simulink model "model_breach"  (R2019b)
settings: Solver=VariableStepAuto  StartTime=0.0  StopTime=nb_time_unit_in_a_simulation/5  RelTol=1e-3
values from neighbouring files (symbols this model uses):
  nb_air_cons = nb_rooms-2    [load_parameters.m]
  nb_boilers = 2    [load_parameters.m]
  nb_radiators = nb_rooms-2    [load_parameters.m]
  nb_second_in_timeunit = 60*5    (= 300)    [full_test.m]
  nb_step_to_fifteen_min = 3    [full_test.m]
  nb_step_to_one_h = 12    [full_test.m]
  nb_step_to_thirty_min = 6    [full_test.m]
  timeunit_in_a_day = 2*6*24    (= 288)    [full_test.m]
undefined symbols (not defined in the file or in its folder): air_mass_kg_rooms, Area_boiler, area_outdoor_rooms, Area_radiators, area_rooms_ground, area_walls_between_rooms, C_air, C_water, Energy_used_by_air_conditioner_for_1_timeunit_in_Watts_vector, Energy_used_by_air_mixer_for_1_timeunit_in_Watts, Energy_used_by_boiler_for_1_timeunit_in_Watts, initial_relative_humidity, initial_temp_water_in_boilers, initial_temperature_rooms, initial_temperature_water_in_radiator, k_boiler_border, k_radiators, k_wall_outdoor_rooms, k_walls_between_rooms, mass_water_radiator, matrix_AC_rooms_locations, matrix_boiler_radiator_connection, matrix_boiler_rooms_locations, matrix_radiator_rooms_locations, nb_humans, nb_rooms, outdoor_max_temp_A, outdoor_max_temp_B, outdoor_min_temp_A, outdoor_min_temp_B, tau_boiler, thickness_boiler, thickness_outdoor_rooms, thickness_radiator_pipes, thickness_walls_between_rooms, Volume_radiators, Volume_rooms, water_weight_in_boiler, watt_generation_of_employe
libraries: dspmtrx3 x15, slstlib x6, dspstat3 x6, simulink x2
(part 2 of 2)

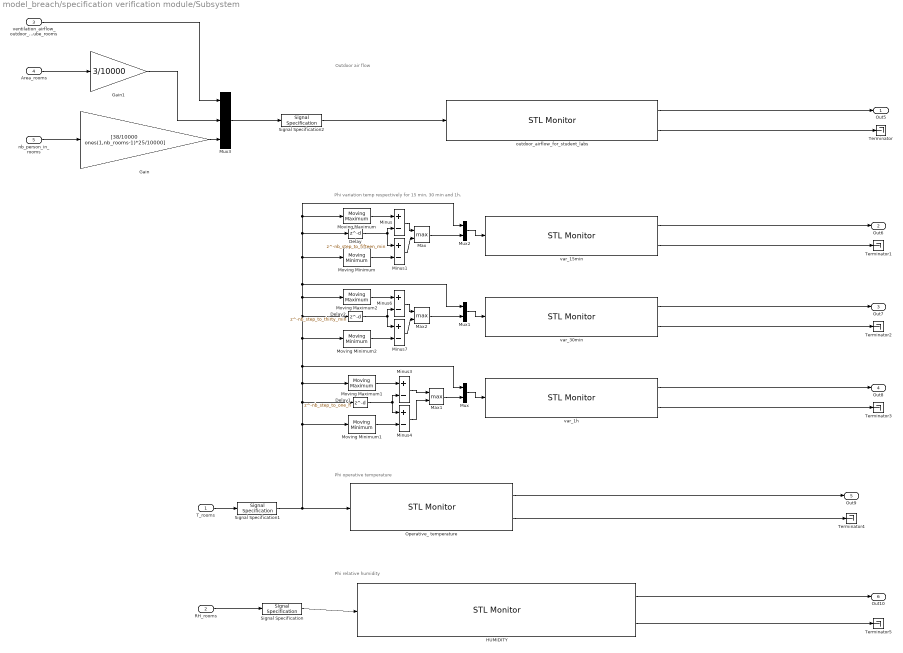
== system model_breach/specification verification module/Subsystem ==
  note: Phi variation temp respectively for 15 min, 30 min and 1h.
  note: Outdoor air flow
  note: Phi operative temperature
  note: Phi relative humidity
  T_rooms : Inport  PortDimensions=nb_rooms
  RH_rooms : Inport  Port=2  PortDimensions=nb_rooms
  ventilation_airflow_outdoor_air_mcube_rooms : Inport  Port=3  PortDimensions=nb_rooms
  Area_rooms : Inport  Port=4  PortDimensions=nb_rooms
  nb_person_in_rooms : Inport  Port=5  OutDataTypeStr=double  PortDimensions=nb_rooms
  Delay : Delay  DelayLength=nb_step_to_fifteen_min  InitialCondition=27
  Delay1 : Delay  DelayLength=nb_step_to_one_h  InitialCondition=27
  Delay2 : Delay  DelayLength=nb_step_to_thirty_min  InitialCondition=27
  Gain : Gain  Gain=[38/10000 ones(1,nb_rooms-1)*25/10000]
  Gain1 : Gain  Gain=3/10000
  "HUMIDITY " : slstlib/STL Monitor  SignalNames=name_rh  STLString=formula_rh  MaxRob=1  RefreshRate=rate  rob_low_lim=inf  rob_up_lim=-inf  rob_diff_lim=-inf
      settings: SourceProductName=Breach Library
  Max : MinMax  Function=max  Inputs=2  ZeroCross=off
  Max1 : MinMax  Function=max  Inputs=2  ZeroCross=off
  Max2 : MinMax  Function=max  Inputs=2  ZeroCross=off
  Minus{,1,3..4,6..7} (6 alike) : Sum  Inputs=+-
  Moving Maximum : dspstat3/Moving Maximum  SpecifyWindowLength=on  WindowLength=nb_step_to_fifteen_min  SimulateUsing=Code generation
      settings: SourceProductName=DSP System Toolbox  SourceProductBaseCode=DS
  Moving Maximum1 : dspstat3/Moving Maximum  SpecifyWindowLength=on  WindowLength=nb_step_to_one_h  SimulateUsing=Code generation
      settings: SourceProductName=DSP System Toolbox  SourceProductBaseCode=DS
  Moving Maximum2 : dspstat3/Moving Maximum  SpecifyWindowLength=on  WindowLength=nb_step_to_thirty_min  SimulateUsing=Code generation
      settings: SourceProductName=DSP System Toolbox  SourceProductBaseCode=DS
  Moving Minimum : dspstat3/Moving Minimum  SpecifyWindowLength=on  WindowLength=nb_step_to_fifteen_min  SimulateUsing=Code generation
      settings: SourceProductName=DSP System Toolbox  SourceProductBaseCode=DS
  Moving Minimum1 : dspstat3/Moving Minimum  SpecifyWindowLength=on  WindowLength=nb_step_to_one_h  SimulateUsing=Code generation
      settings: SourceProductName=DSP System Toolbox  SourceProductBaseCode=DS
  Moving Minimum2 : dspstat3/Moving Minimum  SpecifyWindowLength=on  WindowLength=nb_step_to_thirty_min  SimulateUsing=Code generation
      settings: SourceProductName=DSP System Toolbox  SourceProductBaseCode=DS
  Mux : Mux  Inputs=2
  Mux1 : Mux  Inputs=2
  Mux2 : Mux  Inputs=2
  Mux3 : Mux  Inputs=[nb_rooms nb_rooms nb_rooms]
  Operative_ temperature : slstlib/STL Monitor  SignalNames=name_op_temp  STLString=formula_op_temp  MaxRob=40  RefreshRate=rate  rob_low_lim=inf  rob_up_lim=-inf  rob_diff_lim=-inf
      settings: SourceProductName=Breach Library
  Signal Specification : SignalSpecification  OutMin=-0.25  OutMax=1.25  Dimensions=nb_rooms
  Signal Specification1 : SignalSpecification  OutMin=-100  OutMax=100  Dimensions=nb_rooms
  Signal Specification2 : SignalSpecification  OutMin=-10000  OutMax=10000  Dimensions=nb_rooms*3
  Terminator{,1..5} (6 alike) : Terminator
  outdoor_airflow_for_student_labs : slstlib/STL Monitor  SignalNames=name_out_airflow  STLString=formula_out_airflow  MaxRob=40  RefreshRate=rate  rob_low_lim=inf  rob_up_lim=-inf  rob_diff_lim=-inf
      settings: SourceProductName=Breach Library
  var_15min : slstlib/STL Monitor  SignalNames=name_variation  STLString=formula_fifteen_min_var  MaxRob=2  RefreshRate=rate  rob_low_lim=inf  rob_up_lim=-inf  rob_diff_lim=-inf
      settings: SourceProductName=Breach Library
  var_1h : slstlib/STL Monitor  SignalNames=name_variation  STLString=formula_one_h_var  MaxRob=2  RefreshRate=rate  rob_low_lim=inf  rob_up_lim=-inf  rob_diff_lim=-inf
      settings: SourceProductName=Breach Library
  var_30min : slstlib/STL Monitor  SignalNames=name_variation  STLString=formula_thirty_min_var  MaxRob=2  RefreshRate=rate  rob_low_lim=inf  rob_up_lim=-inf  rob_diff_lim=-inf
      settings: SourceProductName=Breach Library
  Out5 : Outport
  Out6 : Outport  Port=2
  Out7 : Outport  Port=3
  Out8 : Outport  Port=4
  Out9 : Outport  Port=5
  Out10 : Outport  Port=6
  wires:
  Minus1/1 -> Max/2
  Signal Specification1/1 -> Delay1/1, Mux/1, Mux1/1, Delay/1, Mux2/1, Moving Maximum/1, Moving Minimum/1, Moving Maximum2/1, Delay2/1, Moving Minimum2/1, Moving Maximum1/1, Moving Minimum1/1, Operative_ temperature/1
  Minus/1 -> Max/1
  Max/1 -> Mux2/2
  Signal Specification2/1 -> outdoor_airflow_for_student_labs/1
  Mux2/1 -> var_15min/1
  ventilation_airflow_outdoor_air_mcube_rooms/1 -> Mux3/1
  var_1h/1 -> Out8/1
  Signal Specification/1 -> "HUMIDITY "/1
  Max2/1 -> Mux1/2
  Minus6/1 -> Max2/1
  Minus7/1 -> Max2/2
  Moving Maximum2/1 -> Minus6/1
  Delay/1 -> Minus1/1, Minus/2
  Moving Maximum1/1 -> Minus3/1
  Moving Minimum1/1 -> Minus4/2
  RH_rooms/1 -> Signal Specification/1
  Delay2/1 -> Minus6/2, Minus7/1
  Minus3/1 -> Max1/1
  Moving Minimum/1 -> Minus1/2
  Gain1/1 -> Mux3/2
  Mux/1 -> var_1h/1
  T_rooms/1 -> Signal Specification1/1
  Operative_ temperature/2 -> Terminator4/1
  Delay1/1 -> Minus3/2, Minus4/1
  Max1/1 -> Mux/2
  Minus4/1 -> Max1/2
  Area_rooms/1 -> Gain1/1
  Mux1/1 -> var_30min/1
  Gain/1 -> Mux3/3
  "HUMIDITY "/2 -> Terminator5/1
  Moving Maximum/1 -> Minus/1
  nb_person_in_rooms/1 -> Gain/1
  var_1h/2 -> Terminator3/1
  var_30min/2 -> Terminator2/1
  var_30min/1 -> Out7/1
  "HUMIDITY "/1 -> Out10/1
  Operative_ temperature/1 -> Out9/1
  var_15min/1 -> Out6/1
  outdoor_airflow_for_student_labs/1 -> Out5/1
  Mux3/1 -> Signal Specification2/1
  Moving Minimum2/1 -> Minus7/2
  outdoor_airflow_for_student_labs/2 -> Terminator/1
  var_15min/2 -> Terminator1/1

== system model_breach/Physical model/Wall heat Exchange module/Value heat exchange outdoor -> rooms ==
  T_rooms : Inport
  outdoor : Inport  Port=2
  Gain : Gain  Gain=area_outdoor_rooms
  Gain1 : Gain  Gain=k_wall_outdoor_rooms
  Gain2 : Gain  Gain=ones(nb_rooms,1)./thickness_outdoor_rooms
  Sum : Sum  Inputs=|+-
  Q_outdoor_to_rooms : Outport
  wires:
  T_rooms/1 -> Sum/2
  outdoor/1 -> Sum/1
  Sum/1 -> Gain/1
  Gain/1 -> Gain1/1
  Gain1/1 -> Gain2/1
  Gain2/1 -> Q_outdoor_to_rooms/1

== system model_breach/Physical model/Wall heat Exchange module/Value heat exchange within building ==
  "T_rooms " : Inport
  Constant : Constant  Value=diag(ones(nb_rooms,1))
  Gain3 : Gain  Gain=area_walls_between_rooms
  Gain4 : Gain  Gain=k_walls_between_rooms
  Gain8 : Gain  Gain=ones(nb_rooms,nb_rooms)./thickness_walls_between_rooms
  MATRIX WITH ROOM TEMPERATURE DIFFERENCE The area matrix after handles the case of non-adjacent rooms : dspmtrx3/Array-Vector Multiply  mode=Mute  saveAsFlag=0  Dimension=2  V_Source=Input port  V_VectFromMask=[0.5 0.25]  roundingMode=Floor  overflowMode=off  firstCoeffSignedness=Auto  firstCoeffDataTypeStr=Inherit: Same word length as input  firstCoeffMin=[]  firstCoeffMax=[]  firstCoeffLastDataTypeStr=Inherit: Same word length as input  prodOutputSignedness=Auto  accumSignedness=Auto  outputSignedness=Auto  outputDataTypeStr=Inherit: Same as product output  outputMin=[]  outputMax=[]  outputLastDataTypeStr=Inherit: Same as product output
      settings: SourceProductName=DSP System Toolbox  SourceProductBaseCode=DS
  Sum of Elements : Sum  Inputs=+  CollapseMode=Specified dimension  CollapseDim=2
  Q_in_building_to_rooms : Outport
  wires:
  Gain4/1 -> Gain8/1
  Gain3/1 -> Gain4/1
  MATRIX WITH ROOM TEMPERATURE DIFFERENCE The area matrix after handles the case of non-adjacent rooms/1 -> Gain3/1
  Gain8/1 -> Sum of Elements/1
  Sum of Elements/1 -> Q_in_building_to_rooms/1
  Constant/1 -> MATRIX WITH ROOM TEMPERATURE DIFFERENCE The area matrix after handles the case of non-adjacent rooms/1
  "T_rooms "/1 -> MATRIX WITH ROOM TEMPERATURE DIFFERENCE The area matrix after handles the case of non-adjacent rooms/2
